simulink model "DCM_Pulse_Converter"  (R2025a)
settings: Solver=ode5  StartTime=0.0  StopTime=t_end  FixedStep=dt  RelTol=1e-3  EnableMultiTasking=on
values from neighbouring files (symbols this model uses):
  dt = 1e-5    (= 1e-05)    [Experiment_1_DCM_Parameter.m]
  L_A = 374e-3    (= 0.374)    [Experiment_1_DCM_Parameter.m]
  R_A = 22    [Experiment_1_DCM_Parameter.m]
  T_c = 1/1000    (= 0.001)    [Experiment_1_DCM_Parameter.m]
libraries: spsIGBTDiodeLib x4, spsDCVoltageSourceLib x2, simulink x1, spsCurrentMeasurementLib x1, spsSeriesRLCBranchLib x1, spsVoltageMeasurementLib x1, sps_lib x1
settings Model: Creator=BinLi  LastModifiedBy=lucaslee
settings SolverCC: AlgebraicLoopSolver=TrustRegion
settings DataIOCC: LimitDataPoints=on  SaveFormat=Array  SignalLoggingSaveFormat=ModelDataLogs  ReturnWorkspaceOutputs=off
settings OptimizationCC: ExpressionDepthLimit=2147483647.0  LifeSpan=inf
settings DebuggingCC: UnderspecifiedInitializationDetection=Classic  MergeDetectMultiDrivingBlocksExec=none  SolverPrmCheckMsg=warning  FcnCallInpInsideContextMsg=warning  UnconnectedInputMsg=warning  UnconnectedOutputMsg=warning  UnconnectedLineMsg=warning  StateNameClashWarn=warning  SFUnexpectedBacktrackingDiag=warning  SFNoUnconditionalDefaultTransitionDiag=warning  SFExecutionAtInitializationDiag=none  ArithmeticOperatorsInVariantConditions=warning
settings HardwareCC: ProdBitPerPointer=32.0  ProdBitPerSizeT=32.0  ProdBitPerPtrDiffT=32.0  ProdLargestAtomicFloat=None  ProdIntDivRoundTo=Undefined  ProdEndianess=Unspecified  ProdWordSize=32.0  ProdHWDeviceType=32-bit Generic
settings ModelReferenceCC: EnableRefExpFcnMdlSchedulingChecks=on  PropagateSignalLabelsOutOfModel=off
settings SFSimCC: SimUseLocalCustomCode=off  CustomCodeUndefinedFunction=UseInterfaceOnly
settings RTWCC: RTWUseLocalCustomCode=off  GPUComputeCapability=3.5
settings CodeAppCC: StateflowObjectComments=on
settings GRTTargetCC: TargetLangStandard=C89/C90 (ANSI)  CombineOutputUpdateFcns=off  GRTInterface=on
settings ConfigComp: CovMetricSettings=dw  CovSaveCumulativeToWorkspaceVar=on  CovSaveSingleToWorkspaceVar=on  CovExternalEMLEnable=off  CovSFcnEnable=off
settings SimscapeCC: SimscapeNormalizeSystem=off
settings ConfigurationSet: Description=SimMechanics 2G

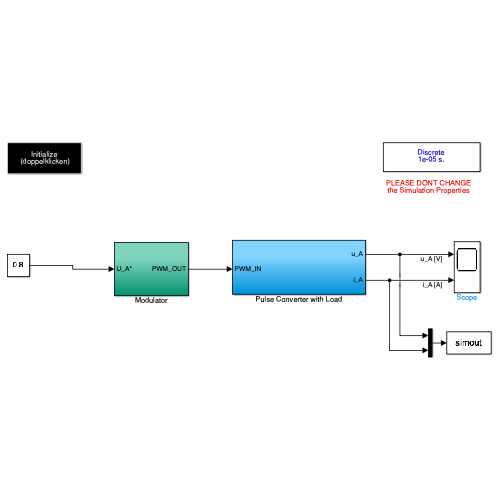
[thumbnail: Simulink's stored preview of the top-level diagram]
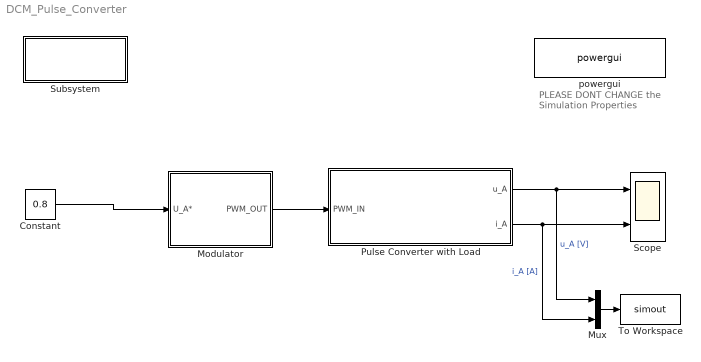
== system DCM_Pulse_Converter ==
  note: PLEASE DONT CHANGE
      | the Simulation Properties
  Constant : Constant  Value=0.8
  Modulator : Subsystem
  Mux : Mux  Inputs=2
  Pulse Converter with Load : Subsystem
  Scope : Scope  NumInputPorts=2
      settings: ActiveDisplayYMinimum=-275.00026333165351  ActiveDisplayYMaximum=275.00256623076228
  Subsystem : Subsystem
      settings: OpenFcn=Experiment_1_DCM_Parameter
      mask Display: disp('Initialize\n (doppelklicken)')
  To Workspace : ToWorkspace  VariableName=simout  SaveFormat=Structure With Time  SampleTime=-1
  powergui : sps_lib/powergui  Priority=1  SimulationMode=Discrete  SampleTime=dt  frequency=60  Iterations=50  frequencyindice=0  Pbase=100e6  ErrMax=1e-4  UnitsV=kV  UnitsW=MW  buscounter=0  FunctionMessages=off  echomessages=off  EnableUseOfTLC=off  CurrentSourceSwitches=off  DisableSnubberDevices=off  DisableRonSwitches=off  DisableVfSwitches=off  DisplayEquations=off  AutomaticDiscreteSolvers=off  SolverType=Tustin  Interpol=off  ExternalGateDelay=off  methode=off  Ts=0  x0status=blocks  SPID=off  SwTol=0  HookPort=off  NonlinearTolerance=1e-4  nMaxIteration=100  ContinueOnMaxIteration=off  RestoreLinks=warning  ResistiveCurrentMeasurement=off  Frange=[0:2:500]  Ylog=off  Xlog=on  ShowGrid=off  save=off  variable=ZData  structure=0  ZoomFFT=off  StartTime=0.0  cycles=1  DisplayStyle=1  fundamental=60  FreqAxis=off  MaxFrequency=1000  frequencyindicesteady=1  RmsSteady=1  display=off
  wires:
  Modulator/1(PWM_OUT) -> Pulse Converter with Load/1(PWM_IN)
  Pulse Converter with Load/1(u_A) -> Mux/1, Scope/1  "u_A [V]"
  Pulse Converter with Load/2(i_A) -> Mux/2, Scope/2  "i_A [A]"
  Mux/1 -> To Workspace/1
  Constant/1 -> Modulator/1(U_A*)

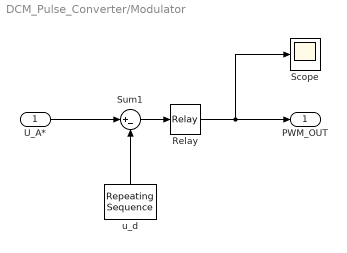
== system DCM_Pulse_Converter/Modulator ==
  U_A* : Inport
  Relay : Relay  OnSwitchValue=1e-4  OffSwitchValue=-1e-4
  Scope : Scope
      settings: ActiveDisplayYMinimum=-10.05524861878453  ActiveDisplayYMaximum=9.94475138121547
  Sum1 : Sum  Inputs=|+-
  u_d : simulink/Sources/Repeating Sequence  rep_seq_t=[0 T_c/2 T_c ]  rep_seq_y=[1 -1 1]
  PWM_OUT : Outport
  wires:
  u_d/1 -> Sum1/2
  Sum1/1 -> Relay/1
  Relay/1 -> Scope/1, PWM_OUT/1
  U_A*/1 -> Sum1/1

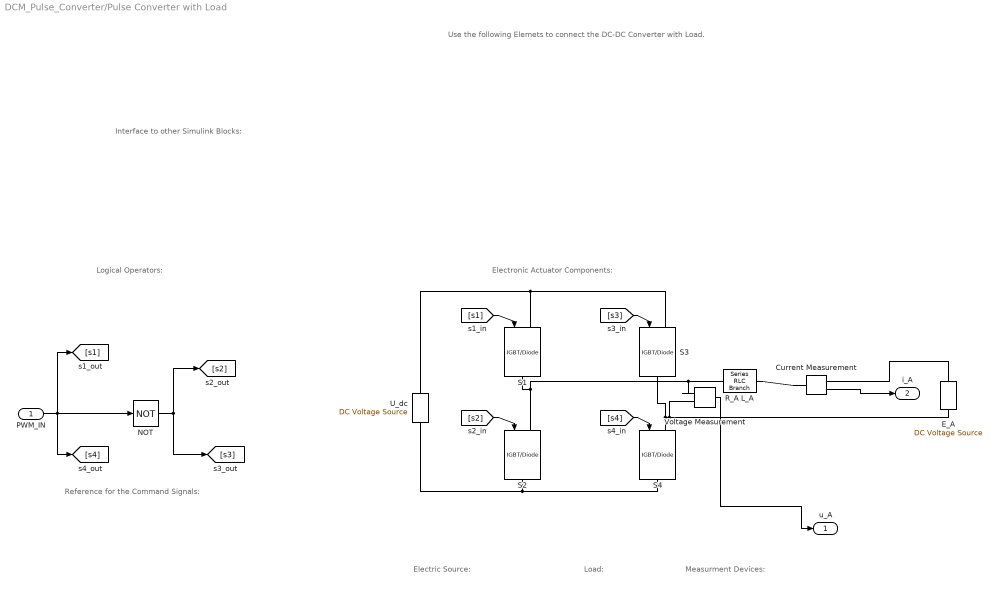
== system DCM_Pulse_Converter/Pulse Converter with Load ==
  note: Use the following Elemets to connect the
      | DC-DC Converter with Load.
  note: Electric Source:
  note: Reference for the Command Signals:
  note: Electronic Actuator Components:
  note: Load:
  note: Logical Operators:
  note: Measurment Devices:
  note: Interface to other Simulink Blocks:
  PWM_IN : Inport
  Current Measurement : spsCurrentMeasurementLib/Current Measurement  PhasorSimulation=off  OutputType=Complex  PSBequivalent=0
  E_A : spsDCVoltageSourceLib/DC Voltage Source  Amplitude=200  Measurements=None
  NOT : Logic  Operator=NOT  AllPortsSameDT=off  OutDataTypeStr=boolean
  R_A L_A : spsSeriesRLCBranchLib/Series RLC Branch  LConnTagsString=__new0  RConnTagsString=__new0  BranchType=RL  Resistance=R_A  Inductance=L_A  SetiL0=off  InitialCurrent=0  Capacitance=[]  Setx0=off  InitialVoltage=0  Measurements=None
  S{1..4} (4 alike) : spsIGBTDiodeLib/IGBT//Diode  Ron=1e-3  Rs=1e5  Cs=inf  Measurements=off
  U_dc : spsDCVoltageSourceLib/DC Voltage Source  Amplitude=220  Measurements=None
  Voltage Measurement : spsVoltageMeasurementLib/Voltage Measurement  Tag=PoWeRsYsTeMmEaSuReMeNt  PhasorSimulation=off  OutputType=Magnitude  PSBequivalent=0
  u_A : Outport
  i_A : Outport  Port=2
  wires:
  [s4] -> S4/1
  [s3] -> S3/1
  [s1] -> S1/1
  [s2] -> S2/1
  Voltage Measurement/1 -> u_A/1
  Current Measurement/1 -> i_A/1
  PWM_IN/1 -> [s4], NOT/1, [s1]
  NOT/1 -> [s2], [s3]
  connections:
  U_dc/RConn1 -- S3/LConn1 -- S1/LConn1
  U_dc/LConn1 -- S4/RConn1 -- S2/RConn1
  S1/RConn1 -- S2/LConn1 -- Voltage Measurement/LConn1 -- R_A L_A/LConn1
  S3/RConn1 -- E_A/LConn1 -- Voltage Measurement/LConn2 -- S4/LConn1
  E_A/RConn1 -- Current Measurement/RConn1
  Current Measurement/LConn1 -- R_A L_A/RConn1

== system DCM_Pulse_Converter/Subsystem ==
